simulink model "Project1SimForced"  (R2013a)
settings: Solver=ode3  StartTime=0.0  StopTime=30  FixedStep=.1  RelTol=1e-3
values from neighbouring files (symbols this model uses):
  c1 = 1    [oscnonlinear.m]    (also in project1.m; project1ODElinear.m; project1nonlinear.m; week1.m)
  c2 = 2    [oscnonlinear.m]    (also in project1.m; project1ODElinear.m; project1nonlinear.m; week1.m)
  k1 = 5    [oscnonlinear.m]    (also in project1.m = 2; project1ODElinear.m; project1nonlinear.m; week1.m = 2)
  k2 = .2    (= 0.2)    [oscnonlinear.m]    (also in project1.m; project1ODElinear.m; project1nonlinear.m; week1.m)
  m1 = 2    [oscnonlinear.m]    (also in project1.m; project1ODElinear.m; project1nonlinear.m; week1.m)
  m2 = 1    [oscnonlinear.m]    (also in project1.m; project1ODElinear.m; project1nonlinear.m; week1.m)
settings Model: Creator=z  LastModifiedBy=z

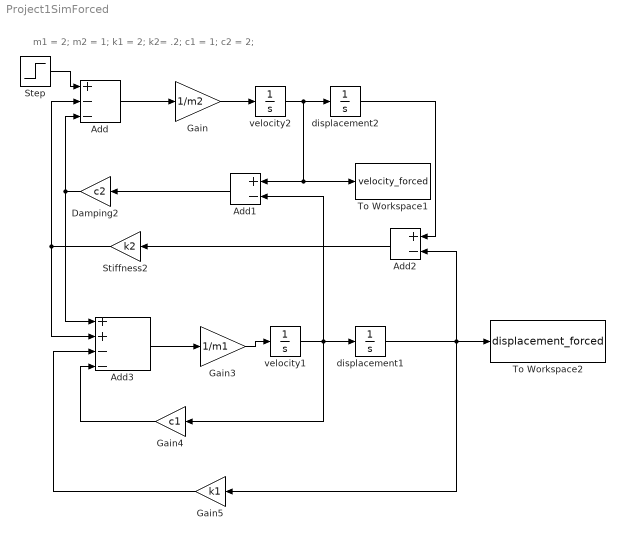
== system Project1SimForced ==
  note: m1 = 2; m2 = 1; k1 = 2; k2= .2; c1 = 1; c2 = 2;
  Add : Sum  Inputs=+--
  Add1 : Sum  Inputs=+-
  Add2 : Sum  Inputs=+-
  Add3 : Sum  Inputs=++--
  Damping2 : Gain  Gain=c2
  Gain : Gain  Gain=1/m2
  Gain3 : Gain  Gain=1/m1
  Gain4 : Gain  Gain=c1
  Gain5 : Gain  Gain=k1
  Step : Step  Time=0  SampleTime=0
  "Stiffness2 " : Gain  Gain=k2
  To Workspace1 : ToWorkspace  VariableName=velocity_forced  SampleTime=-1  SaveFormat=Timeseries
  To Workspace2 : ToWorkspace  VariableName=displacement_forced  SampleTime=-1  SaveFormat=Timeseries
  "displacement1 " : Integrator
  displacement2 : Integrator
  "velocity1 " : Integrator
  velocity2 : Integrator
  wires:
  Add/1 -> Gain/1
  Gain/1 -> velocity2/1
  velocity2/1 -> To Workspace1/1, Add1/1, displacement2/1
  displacement2/1 -> Add2/1
  Add2/1 -> "Stiffness2 "/1
  Add1/1 -> Damping2/1
  Damping2/1 -> Add3/1, Add/3
  "Stiffness2 "/1 -> Add/2, Add3/2
  Add3/1 -> Gain3/1
  Gain3/1 -> "velocity1 "/1
  "velocity1 "/1 -> Add1/2, Gain4/1, "displacement1 "/1
  "displacement1 "/1 -> To Workspace2/1, Add2/2, Gain5/1
  Gain4/1 -> Add3/4
  Gain5/1 -> Add3/3
  Step/1 -> Add/1
